simulink model "PX4_to_sim"  (R2018b)
settings: Solver=VariableStepAuto  StartTime=0.0  StopTime=inf  RelTol=1e-3
undefined symbols (not defined in the file or in its folder): serial
libraries: aerolibutil x2, instrumentlib x2, vrlib x1
settings Model: Creator=Robert  LastModifiedBy=Robert

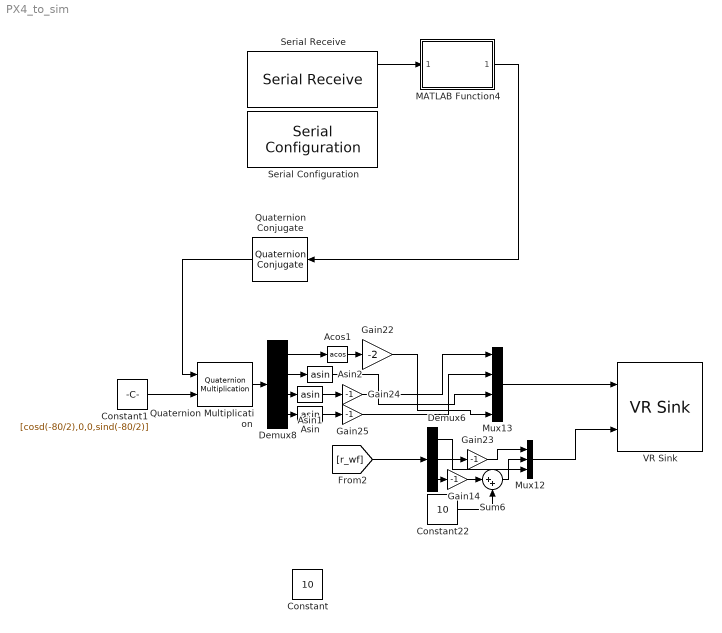
== system PX4_to_sim ==
  Acos1 : Trigonometry  Operator=acos
  Asin : Trigonometry  Operator=asin
  Asin1 : Trigonometry  Operator=asin
  Asin2 : Trigonometry  Operator=asin
  Constant : Constant  Value=10
  Constant1 : Constant  Value=[cosd(-80/2),0,0,sind(-80/2)]
  Constant22 : Constant  Value=10
  Demux6 : Demux  Outputs=3
  Demux8 : Demux
  Gain{14,23..25} (4 alike) : Gain  Gain=-1
  Gain22 : Gain  Gain=-2
  MATLAB Function4 : MATLAB Function  TreatAsAtomicUnit=on
  Mux12 : Mux  Inputs=3
  Mux13 : Mux
  Quaternion Conjugate : aerolibutil/Quaternion Conjugate
      settings: SourceProductName=Aerospace Blockset  SourceProductBaseCode=AE
  Quaternion Multiplication : aerolibutil/Quaternion Multiplication
  Serial Configuration : instrumentlib/Serial Configuration  Priority=-200000  ComPortMenu=COM3  ComPort=COM3  ObjConstructor=serial('COM3');  BaudRate=115200  DataBits=8  Parity=none  StopBits=1  FlowControl=none  Timeout=1  ByteOrder=LittleEndian
  Serial Receive : instrumentlib/Serial Receive  ComPortMenu=COM3  ComPort=COM3  ObjConstructor=serial('COM3');  Header=A  Terminator=<none>  DataSize="[1  16]"  DataType=uint8  EnableBlockingMode=off  ActionDataUnavailable=Output last received value  CustomValue=0  SampleTime=0.01
  Sum6 : Sum  Inputs=|++
  VR Sink : vrlib/VR Sink  InstantiateOnLoad=on  SampleTime=0.05  ViewEnable=on  RemoteChange=off  RemoteView=off  FieldsWritten=Plane.rotation.4.1.1.double#Plane.translation.3.1.1.double  WorldFileName=vrtkoff_hud.wrl  WorldDescription=VR Plane Take-Off with HUD Text  AutoView=on  VideoDimensions=[600 860]  AllowVariableSize=off  FigureProperties="{'Position', 'Name', 'Viewpoint', 'CameraBound', 'CameraDirection', 'CameraPosition', 'CameraUpVector', 'ZoomFactor', 'Antialiasing', 'Headlight', 'Lighting', 'NavPanel', 'Sound', 'StatusBar', 'Stereo3D', 'Stereo3DCameraOffset', 'Stereo3DHIT', 'ToolBar', 'Textures', 'Transparency', 'Triad', 'Wireframe', 'NavZones', 'NavMode', 'NavSpeed', 'CaptureFileFormat', 'CaptureFileName', 'Record2DCompressMethod', 'Record2DCompressQuality', 'Record2D', 'Record2DFileName', 'Record2DFPS'; [9.6200000000000000e+02   8.4000000000000000e+01   9.5800000000000000e+02   9.0400000000000000e+02], 'VR Plane Take-Off with HUD Text', 'Observe Plane', 'on', [5.7099446309840346e-02  -3.2219828231407860e-01   9.4494863358012704e-01], [-3.1309971024241530e+00   6.5179831365447862e+00  -2.5311554927991292e+01], [8.3623147595487442e-03   9.4661398615939485e-01   3.2226081502299642e-01], [1.0000000000000000e+00], 'off', 'on', 'on', 'halfbar', 'off', 'on', 'off', [1.0000000149011612e-01], [0.0000000000000000e+00], 'on', 'on', 'on', 'none', 'off', 'on', 'fly', 'normal', 'png', '%f_anim_%n.png', 'auto', [7.5000000000000000e+01], 'on', '%f_anim_%n.avi', 'auto'}"
      settings: SourceProductBaseCode=VR
  wires:
  Serial Receive/1 -> MATLAB Function4/1(data_u8)
  MATLAB Function4/1(singles) -> Quaternion Conjugate/1
  Asin1/1 -> Gain24/1
  Demux6/3 -> Gain14/1
  Gain24/1 -> Mux13/1
  Constant22/1 -> Sum6/2
  Asin/1 -> Gain25/1
  Demux8/2 -> Asin2/1
  Asin2/1 -> Mux13/3
  Gain22/1 -> Mux13/4
  Demux8/1 -> Acos1/1
  Acos1/1 -> Gain22/1
  Demux8/4 -> Asin/1
  [r_wf] -> Demux6/1
  Sum6/1 -> Mux12/2
  Gain14/1 -> Sum6/1
  Demux6/2 -> Gain23/1
  Demux6/1 -> Mux12/3
  Gain25/1 -> Mux13/2
  Demux8/3 -> Asin1/1
  Gain23/1 -> Mux12/1
  Mux13/1 -> VR Sink/1
  Mux12/1 -> VR Sink/2
  Quaternion Multiplication/1 -> Demux8/1
  Constant1/1 -> Quaternion Multiplication/2
  Quaternion Conjugate/1 -> Quaternion Multiplication/1

== matlab function PX4_to_sim/MATLAB Function4 ==
  data: data_u8 input; singles output
function singles = bytes2singles(data_u8)

singles = single(zeros(1,4));
singles = typecast(uint8(data_u8),'single');
